simulink model "c6mdde2"  (Simulink 5.1)
settings: Solver=ode45  StartTime=0.0  StopTime=10.0  RelTol=1e-3
settings Model: LastModifiedBy=tf  BooleanDataType=on  ProdHWDeviceType=Microprocessor

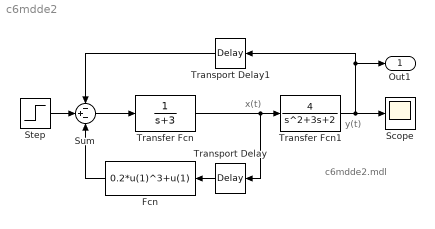
== system c6mdde2 ==
  note: c6mdde2.mdl
  note: x(t)
  note: y(t)
  Fcn : Fcn  Orientation=left  Expr=0.2*u(1)^3+u(1)
  Scope : Scope
      settings: TimeRange=10  YMin=-0.00744048  YMax=0.429067  SaveName=a
  Step : Step  Time=0  SampleTime=0
  Sum : Sum  Inputs=-+-  SaturateOnIntegerOverflow=on
  Transfer Fcn : TransferFcn  Denominator=[1 3]
  Transfer Fcn1 : TransferFcn  Numerator=4  Denominator=[1 3 2]
  Transport Delay : TransportDelay  Orientation=left  DelayTime=0.5
  Transport Delay1 : TransportDelay  Orientation=left
  Out1 : Outport
  wires:
  Transfer Fcn/1 -> Transfer Fcn1/1, Transport Delay/1
  Transfer Fcn1/1 -> Scope/1, Transport Delay1/1, Out1/1
  Transport Delay/1 -> Fcn/1
  Sum/1 -> Transfer Fcn/1
  Fcn/1 -> Sum/3
  Step/1 -> Sum/2
  Transport Delay1/1 -> Sum/1
